simulink model "machine_x"  (R2026a)
settings: Solver=FixedStepAuto  FixedStep=0.0001
values from neighbouring files (symbols this model uses):
  c_a = 50    [init_params.m]
  c_x = 500    [init_params.m]
  k_c = 1e5    (= 100000)    [init_params.m]
libraries: fl_lib x31, nesl_utility x15, sdl_lib x1
settings Model: Creator=leo  LastModifiedBy=leo
settings SimscapeCC: SimscapeNominalValues="[{\"value\":\"1\",\"unit\":\"A\"},{\"value\":\"1\",\"unit\":\"bar\"},{\"value\":\"1\",\"unit\":\"cm^2\"},{\"value\":\"1\",\"unit\":\"cm^3/s\"},{\"value\":\"1\",\"unit\":\"kJ/kg\"},{\"value\":\"1\",\"unit\":\"kW\"},{\"value\":\"1\",\"unit\":\"l\"},{\"value\":\"1\",\"unit\":\"N\"},{\"value\":\"1\",\"unit\":\"N*m\"},{\"value\":\"1\",\"unit\":\"V\"}]"  SimscapeLogType=none  SimscapeLogDataHistory=5000.0

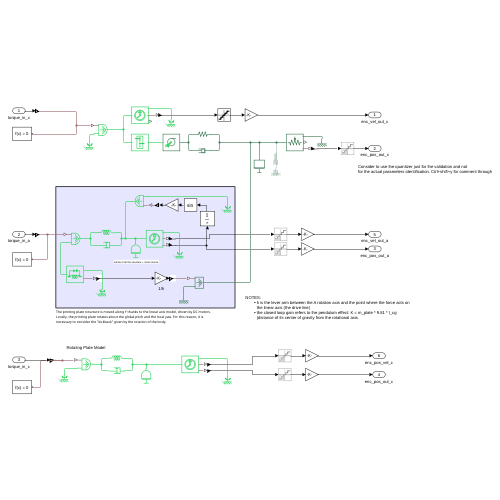
[thumbnail: Simulink's stored preview of the top-level diagram]
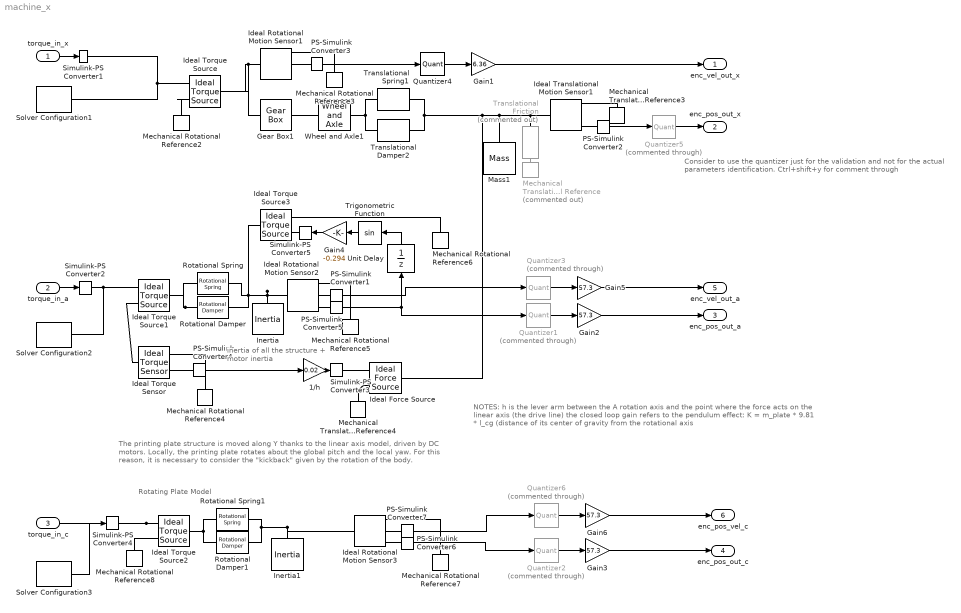
== system machine_x ==
  note: NOTES:
      | h is the lever arm between the A rotation axis and the point where the force acts on the linear axis (the drive line)
      | the closed loop gain refers to the pendulum effect: K = m_plate * 9.81 * l_cg (distance of its center of gravity from the rotational axis
  note: Consider to use the quantizer just for the validation and not
      | for the actual parameters identification. Ctrl+shift+y for comment through
  note: Rotating Plate Model
  note: inertia of all the structure + motor inertia
  note: The printing plate structure is moved along Y thanks to the linear axis model, driven by DC motors.
      | Locally, the printing plate rotates about the global pitch and the local yaw. For this reason, it is necessary to consider the "kickback" given by the rotation of the body.
  torque_in_x : Inport
  torque_in_a : Inport  Port=2
  torque_in_c : Inport  Port=3
  1/h : Gain  Gain=0.02
  Gain1 : Gain  Gain=6.36
  Gain{2..3,5..6} (4 alike) : Gain  Gain=57.3
  Gain4 : Gain  Gain=-0.294
  Gear Box1 : fl_lib/Mechanical/Mechanisms/Gear Box  ratio=27  t_in_specify=off  t_in_priority=None  t_in=0 N*m  t_in_nominal_specify=off  t_in_nominal_value=1  t_in_nominal_unit=N*m  t_out_specify=off  t_out_priority=None  t_out=0 N*m  t_out_nominal_specify=off  t_out_nominal_value=1  t_out_nominal_unit=N*m
  Ideal Force Source : fl_lib/Mechanical/Mechanical Sources/Ideal Force Source
  Ideal Rotational Motion Sensor1 : fl_lib/Mechanical/Mechanical Sensors/Ideal Rotational Motion Sensor  reference=foundation.enum.MeasurementReference.difference  acceleration_port=false  velocity_port=true  position_port=true  wrap_angle=false  offset=0 rad
  Ideal Rotational Motion Sensor2 : fl_lib/Mechanical/Mechanical Sensors/Ideal Rotational Motion Sensor  reference=foundation.enum.MeasurementReference.difference  acceleration_port=false  velocity_port=true  position_port=true  wrap_angle=false  offset=0 rad
  Ideal Rotational Motion Sensor3 : fl_lib/Mechanical/Mechanical Sensors/Ideal Rotational Motion Sensor  reference=foundation.enum.MeasurementReference.difference  acceleration_port=false  velocity_port=true  position_port=true  wrap_angle=false  offset=0 rad
  Ideal Torque Sensor : fl_lib/Mechanical/Mechanical Sensors/Ideal Torque Sensor
  Ideal Torque Source{,1..3} (4 alike) : fl_lib/Mechanical/Mechanical Sources/Ideal Torque Source
  Ideal Translational Motion Sensor1 : fl_lib/Mechanical/Mechanical Sensors/Ideal Translational Motion Sensor  reference=foundation.enum.MeasurementReference.difference  acceleration_port=false  velocity_port=true  position_port=true  offset=0 m
  Inertia : fl_lib/Mechanical/Rotational Elements/Inertia  inertia=J_a kg*m^2  num_ports=foundation.enum.numPorts2.one  w_specify=off  w_priority=High  w=0 rad/s  w_nominal_specify=off  w_nominal_value=1  w_nominal_unit=rad/s  t_specify=off  t_priority=None  t=0 N*m  t_nominal_specify=off  t_nominal_value=1  t_nominal_unit=N*m
  Inertia1 : fl_lib/Mechanical/Rotational Elements/Inertia  inertia=J_c kg*m^2  num_ports=foundation.enum.numPorts2.one  w_specify=off  w_priority=High  w=0 rad/s  w_nominal_specify=off  w_nominal_value=1  w_nominal_unit=rad/s  t_specify=off  t_priority=None  t=0 N*m  t_nominal_specify=off  t_nominal_value=1  t_nominal_unit=N*m
  Mass1 : fl_lib/Mechanical/Translational Elements/Mass  mass=m_x kg  num_ports=foundation.enum.numPorts2.one  v_specify=off  v_priority=High  v=0 m/s  v_nominal_specify=off  v_nominal_value=1  v_nominal_unit=m/s  f_specify=off  f_priority=None  f=0 N  f_nominal_specify=off  f_nominal_value=1  f_nominal_unit=N
  Mechanical Rotational Reference{2..8} (7 alike) : fl_lib/Mechanical/Rotational Elements/Mechanical Rotational Reference
  Mechanical Translational Reference : fl_lib/Mechanical/Translational Elements/Mechanical Translational Reference  Commented=on
  Mechanical Translational Reference3 : fl_lib/Mechanical/Translational Elements/Mechanical Translational Reference
  Mechanical Translational Reference4 : fl_lib/Mechanical/Translational Elements/Mechanical Translational Reference
  PS-Simulink Converter{1,4..7} (5 alike) : nesl_utility/PS-Simulink Converter  PhysicalDomain=network_engine_domain  SubClassName=ps_output  LeftPortType=input  RightPortType=output  PseudoPeriodic=off  Frequencies=[]  VectorFormat=inherit  Unit=inherit  AffineConversion=off
  PS-Simulink Converter2 : nesl_utility/PS-Simulink Converter  PhysicalDomain=network_engine_domain  SubClassName=ps_output  LeftPortType=input  RightPortType=output  PseudoPeriodic=off  Frequencies=[]  VectorFormat=inherit  Unit=mm  AffineConversion=off
  PS-Simulink Converter3 : nesl_utility/PS-Simulink Converter  PhysicalDomain=network_engine_domain  SubClassName=ps_output  LeftPortType=input  RightPortType=output  PseudoPeriodic=off  Frequencies=[]  VectorFormat=inherit  Unit=rad/s  AffineConversion=off
  Quantizer{1..3,5..6} (5 alike) : Quantizer  Commented=through  QuantizationInterval=0.001
  Quantizer4 : Quantizer  QuantizationInterval=0.001
  Rotational Damper : fl_lib/Mechanical/Rotational Elements/Rotational Damper  D=c_a N*m*s/rad  w_specify=off  w_priority=None  w=0 rad/s  w_nominal_specify=off  w_nominal_value=1  w_nominal_unit=rad/s  t_specify=off  t_priority=None  t=0 N*m  t_nominal_specify=off  t_nominal_value=1  t_nominal_unit=N*m
  Rotational Damper1 : fl_lib/Mechanical/Rotational Elements/Rotational Damper  D=k_c N*m*s/rad  w_specify=off  w_priority=None  w=0 rad/s  w_nominal_specify=off  w_nominal_value=1  w_nominal_unit=rad/s  t_specify=off  t_priority=None  t=0 N*m  t_nominal_specify=off  t_nominal_value=1  t_nominal_unit=N*m
  Rotational Spring : fl_lib/Mechanical/Rotational Elements/Rotational Spring  spr_rate=k_a N*m/rad  w_specify=off  w_priority=None  w=0 rad/s  w_nominal_specify=off  w_nominal_value=1  w_nominal_unit=rad/s  t_specify=off  t_priority=None  t=0 N*m  t_nominal_specify=off  t_nominal_value=1  t_nominal_unit=N*m  phi_specify=off  phi_priority=High  phi=0 rad  phi_nominal_specify=off  phi_nominal_value=1  phi_nominal_unit=rad
  Rotational Spring1 : fl_lib/Mechanical/Rotational Elements/Rotational Spring  spr_rate=c_c N*m/rad  w_specify=off  w_priority=None  w=0 rad/s  w_nominal_specify=off  w_nominal_value=1  w_nominal_unit=rad/s  t_specify=off  t_priority=None  t=0 N*m  t_nominal_specify=off  t_nominal_value=1  t_nominal_unit=N*m  phi_specify=off  phi_priority=High  phi=0 rad  phi_nominal_specify=off  phi_nominal_value=1  phi_nominal_unit=rad
  Simulink-PS Converter{1,3..5} (4 alike) : nesl_utility/Simulink-PS Converter  PhysicalDomain=network_engine_domain  SubClassName=ps_input  LeftPortType=input  RightPortType=output  PseudoPeriodic=off  Frequencies=[]  NoiseDistribution=none  NoiseParameters=[]  Unit=1  AffineConversion=off  FilteringAndDerivatives=provide  SimscapeFilterOrder=1  InputFilterTimeConstant=0.001  UdotUserProvided=0
  Simulink-PS Converter2 : nesl_utility/Simulink-PS Converter  PhysicalDomain=network_engine_domain  SubClassName=ps_input  LeftPortType=input  RightPortType=output  PseudoPeriodic=off  Frequencies=[]  NoiseDistribution=none  NoiseParameters=[]  Unit=1  AffineConversion=off  FilteringAndDerivatives=provide  SimscapeFilterOrder=1  InputFilterTimeConstant=0.0001  UdotUserProvided=0
  Solver Configuration1 : nesl_utility/Solver Configuration  PhysicalDomain=network_engine_domain  SubClassName=solver  LeftPortType=input  RightPortType=generic  Tones=[]  Harmonics=[]  SimulateNoise=off  Profile=off  UseLocalSampling=off  EnableSwitchedLinearOptims=on  FrequencyDomain=off  UseCCode=off  RelTol=0.001  AbsTol=0.001  MinStep=1e-09  ToWorkspace=off  RevertToSquareIcSolve=off  NumHomotopyIterations=100  PhasorMode=off  PhasorModeNumHarmonics=1  ConsistencySolver=NEWTON_XTOL_AFTER_FTOL  CanonicalOrdering=UNORDERED  OptimizeIntermediates=UNOPTIMIZED  IndexReductionMethod=DerivativeReplacement  DoDC=off  ResidualTolerance=1e-09  ConsistencyTolSource=GLOBAL  ConsistencyAbsTol=0.001  ConsistencyRelTol=0.001  ConsistencyTolFactor=0.001  UseLocalSolver=on  LocalSolverChoice=NE_BACKWARD_EULER_ADVANCER  ResolveIndetEquations=on  FunctionEvalNumThread=1  LocalSolverSampleTime=0.0001  DoFixedCost=off  MaxNonlinIter=3  MaxModeIter=2  ComputeImpulses=off  ImpulseIterations=2  LinearAlgebra=auto  LinearAlgebraNumThread=0  EquationFormulation=NE_TIME_EF  DelaysMemoryBudget=1024  AutomaticFiltering=on  FilteringTimeConstant=0.001  PartitionStorageMethod=AS_NEEDED  PartitionMemoryBudget=1024  PartitionMethod=ROBUST  MultibodyUseLocalSolver=off  MultibodyLocalSolverChoice=ODE1  MultibodyLocalSolverSampleTime=0.001
  Solver Configuration2 : nesl_utility/Solver Configuration  PhysicalDomain=network_engine_domain  SubClassName=solver  LeftPortType=input  RightPortType=generic  Tones=[]  Harmonics=[]  SimulateNoise=off  Profile=off  UseLocalSampling=off  EnableSwitchedLinearOptims=on  FrequencyDomain=off  UseCCode=off  RelTol=0.001  AbsTol=0.001  MinStep=1e-09  ToWorkspace=off  RevertToSquareIcSolve=off  NumHomotopyIterations=100  PhasorMode=off  PhasorModeNumHarmonics=1  ConsistencySolver=NEWTON_XTOL_AFTER_FTOL  CanonicalOrdering=UNORDERED  OptimizeIntermediates=UNOPTIMIZED  IndexReductionMethod=DerivativeReplacement  DoDC=off  ResidualTolerance=1e-09  ConsistencyTolSource=GLOBAL  ConsistencyAbsTol=0.001  ConsistencyRelTol=0.001  ConsistencyTolFactor=0.001  UseLocalSolver=on  LocalSolverChoice=NE_BACKWARD_EULER_ADVANCER  ResolveIndetEquations=on  FunctionEvalNumThread=1  LocalSolverSampleTime=0.0001  DoFixedCost=off  MaxNonlinIter=3  MaxModeIter=2  ComputeImpulses=off  ImpulseIterations=2  LinearAlgebra=auto  LinearAlgebraNumThread=0  EquationFormulation=NE_TIME_EF  DelaysMemoryBudget=1024  AutomaticFiltering=on  FilteringTimeConstant=0.001  PartitionStorageMethod=AS_NEEDED  PartitionMemoryBudget=1024  PartitionMethod=ROBUST  MultibodyUseLocalSolver=off  MultibodyLocalSolverChoice=ODE1  MultibodyLocalSolverSampleTime=0.001
  Solver Configuration3 : nesl_utility/Solver Configuration  PhysicalDomain=network_engine_domain  SubClassName=solver  LeftPortType=input  RightPortType=generic  Tones=[]  Harmonics=[]  SimulateNoise=off  Profile=off  UseLocalSampling=off  EnableSwitchedLinearOptims=on  FrequencyDomain=off  UseCCode=off  RelTol=0.001  AbsTol=0.001  MinStep=1e-09  ToWorkspace=off  RevertToSquareIcSolve=off  NumHomotopyIterations=100  PhasorMode=off  PhasorModeNumHarmonics=1  ConsistencySolver=NEWTON_XTOL_AFTER_FTOL  CanonicalOrdering=UNORDERED  OptimizeIntermediates=UNOPTIMIZED  IndexReductionMethod=DerivativeReplacement  DoDC=off  ResidualTolerance=1e-09  ConsistencyTolSource=GLOBAL  ConsistencyAbsTol=0.001  ConsistencyRelTol=0.001  ConsistencyTolFactor=0.001  UseLocalSolver=on  LocalSolverChoice=NE_BACKWARD_EULER_ADVANCER  ResolveIndetEquations=on  FunctionEvalNumThread=1  LocalSolverSampleTime=0.0001  DoFixedCost=off  MaxNonlinIter=3  MaxModeIter=2  ComputeImpulses=off  ImpulseIterations=2  LinearAlgebra=auto  LinearAlgebraNumThread=0  EquationFormulation=NE_TIME_EF  DelaysMemoryBudget=1024  AutomaticFiltering=on  FilteringTimeConstant=0.001  PartitionStorageMethod=AS_NEEDED  PartitionMemoryBudget=1024  PartitionMethod=ROBUST  MultibodyUseLocalSolver=off  MultibodyLocalSolverChoice=ODE1  MultibodyLocalSolverSampleTime=0.001
  Translational Friction : fl_lib/Mechanical/Translational Elements/Translational Friction  Commented=on  brkwy_frc=Fb_x N  brkwy_vel=0.1 m/s  Col_frc=Fc_x N  visc_coef=bv_x N*s/m  v_specify=off  v_priority=None  v=0 m/s  v_nominal_specify=off  v_nominal_value=1  v_nominal_unit=m/s  f_specify=off  f_priority=None  f=0 N  f_nominal_specify=off  f_nominal_value=1  f_nominal_unit=N
  Translational Damper2 : sdl_lib/Couplings & Drives/Springs & Dampers/Translational Damper  D=c_x N*s/m  thermal_port=simscape.enum.thermaleffects.omit  thermal_mass=50 kJ/K  temperature_specify=off  temperature_priority=High  temperature=300 K  temperature_nominal_specify=off  temperature_nominal_value=1  temperature_nominal_unit=K
  Translational Spring1 : fl_lib/Mechanical/Translational Elements/Translational Spring  spr_rate=k_x N/m  v_specify=off  v_priority=None  v=0 m/s  v_nominal_specify=off  v_nominal_value=1  v_nominal_unit=m/s  f_specify=off  f_priority=None  f=0 N  f_nominal_specify=off  f_nominal_value=1  f_nominal_unit=N  x_specify=off  x_priority=High  x=0 m  x_nominal_specify=off  x_nominal_value=1  x_nominal_unit=m
  Trigonometric Function : Trigonometry
  Unit Delay : UnitDelay  SampleTime=-1
  Wheel and Axle1 : fl_lib/Mechanical/Mechanisms/Wheel and Axle  R=6.36 mm  or=foundation.enum.DriveOrientation.Positive  t_specify=off  t_priority=None  t=0 N*m  t_nominal_specify=off  t_nominal_value=1  t_nominal_unit=N*m  f_specify=off  f_priority=None  f=0 N  f_nominal_specify=off  f_nominal_value=1  f_nominal_unit=N
  enc_vel_out_x : Outport
  enc_pos_out_x : Outport  Port=2
  enc_pos_out_a : Outport  Port=3
  enc_pos_out_c : Outport  Port=4
  enc_vel_out_a : Outport  Port=5
  enc_pos_vel_c : Outport  Port=6
  wires:
  Gain4/1 -> Simulink-PS Converter5/1
  Quantizer5/1 -> enc_pos_out_x/1
  Unit Delay/1 -> Trigonometric Function/1
  Gain2/1 -> enc_pos_out_a/1
  PS-Simulink Converter4/1 -> 1/h/1
  PS-Simulink Converter3/1 -> Quantizer4/1
  PS-Simulink Converter6/1 -> Quantizer2/1
  Quantizer1/1 -> Gain2/1
  Quantizer4/1 -> Gain1/1
  torque_in_x/1 -> Simulink-PS Converter1/1
  Quantizer2/1 -> Gain3/1
  Trigonometric Function/1 -> Gain4/1
  PS-Simulink Converter5/1 -> Quantizer1/1, Unit Delay/1
  torque_in_c/1 -> Simulink-PS Converter4/1
  Gain3/1 -> enc_pos_out_c/1
  Gain1/1 -> enc_vel_out_x/1
  1/h/1 -> Simulink-PS Converter3/1
  torque_in_a/1 -> Simulink-PS Converter2/1
  PS-Simulink Converter2/1 -> Quantizer5/1
  Gain5/1 -> enc_vel_out_a/1
  Quantizer3/1 -> Gain5/1
  PS-Simulink Converter1/1 -> Quantizer3/1
  PS-Simulink Converter7/1 -> Quantizer6/1
  Gain6/1 -> enc_pos_vel_c/1
  Quantizer6/1 -> Gain6/1
  connections:
  Inertia1/LConn1 -- Ideal Rotational Motion Sensor3/LConn1 -- Rotational Damper1/RConn1 -- Rotational Spring1/RConn1
  Ideal Translational Motion Sensor1/LConn1 -- Translational Spring1/RConn1 -- Translational Damper2/RConn1 -- Ideal Force Source/LConn1 -- Mass1/LConn1 -- Translational Friction/LConn1
  Rotational Spring1/LConn1 -- Rotational Damper1/LConn1 -- Ideal Torque Source2/LConn1
  Simulink-PS Converter2/RConn1 -- Solver Configuration2/RConn1 -- Ideal Torque Source1/RConn1
  Rotational Damper/LConn1 -- Rotational Spring/LConn1 -- Ideal Torque Source1/LConn1
  Ideal Rotational Motion Sensor1/LConn1 -- Ideal Torque Source/LConn1 -- Gear Box1/LConn1
  Translational Spring1/LConn1 -- Translational Damper2/LConn1 -- Wheel and Axle1/RConn1
  Inertia/LConn1 -- Ideal Torque Source3/LConn1 -- Rotational Spring/RConn1 -- Rotational Damper/RConn1 -- Ideal Rotational Motion Sensor2/LConn1
  Ideal Torque Source2/RConn1 -- Simulink-PS Converter4/RConn1 -- Solver Configuration3/RConn1
  Solver Configuration1/RConn1 -- Ideal Torque Source/RConn1 -- Simulink-PS Converter1/RConn1
  Ideal Force Source/RConn1 -- Simulink-PS Converter3/RConn1
  Mechanical Rotational Reference6/LConn1 -- Ideal Torque Source3/RConn2
  PS-Simulink Converter5/LConn1 -- Ideal Rotational Motion Sensor2/RConn3
  Ideal Rotational Motion Sensor3/RConn1 -- Mechanical Rotational Reference7/LConn1
  Ideal Rotational Motion Sensor1/RConn1 -- Mechanical Rotational Reference3/LConn1
  Ideal Torque Source3/RConn1 -- Simulink-PS Converter5/RConn1
  Ideal Torque Source1/RConn2 -- Ideal Torque Sensor/LConn1
  Mechanical Rotational Reference8/LConn1 -- Ideal Torque Source2/RConn2
  Mechanical Translational Reference4/LConn1 -- Ideal Force Source/RConn2
  Ideal Rotational Motion Sensor1/RConn2 -- PS-Simulink Converter3/LConn1
  Gear Box1/RConn1 -- Wheel and Axle1/LConn1
  Ideal Rotational Motion Sensor2/RConn1 -- Mechanical Rotational Reference5/LConn1
  PS-Simulink Converter2/LConn1 -- Ideal Translational Motion Sensor1/RConn3
  PS-Simulink Converter6/LConn1 -- Ideal Rotational Motion Sensor3/RConn3
  Ideal Torque Sensor/RConn2 -- PS-Simulink Converter4/LConn1
  Ideal Translational Motion Sensor1/RConn1 -- Mechanical Translational Reference3/LConn1
  Ideal Torque Source/RConn2 -- Mechanical Rotational Reference2/LConn1
  Ideal Torque Sensor/RConn1 -- Mechanical Rotational Reference4/LConn1
  PS-Simulink Converter1/LConn1 -- Ideal Rotational Motion Sensor2/RConn2
  PS-Simulink Converter7/LConn1 -- Ideal Rotational Motion Sensor3/RConn2
  Mechanical Translational Reference/LConn1 -- Translational Friction/RConn1
